simulink model "reaktor"  (R2016a)
settings: Solver=VariableStepAuto  StartTime=0.0  StopTime=100  RelTol=1e-3
values from neighbouring files (symbols this model uses):
  A_fm = 59900/3    (= 19966.6666667)    [zmienne.m]
  alfa_c = -2.0 * 10^-4    (= -0.0002)    [zmienne.m]
  alfa_f = -1.1 * 10^-5    (= -1.1e-05)    [zmienne.m]
  B_1 = 0.000209    [zmienne.m]
  B_2 = 0.001414    [zmienne.m]
  B_3 = 0.001309    [zmienne.m]
  B_4 = 0.002727    [zmienne.m]
  B_5 = 0.000925    [zmienne.m]
  B_6 = 0.000314    [zmienne.m]
  B_t = 0.00689    [zmienne.m]
  C_pf = 0.059    [zmienne.m]
  C_pmo = 1.39    [zmienne.m]
  CP_fw = 1.218    [zmienne.m]
  F_r = 0.974    [zmienne.m]
  H_fm = 200/3600    (= 0.0555555555556)    [zmienne.m]
  K9 = -0.035    [zmienne.m]
  lambda_1 = 0.0125    [zmienne.m]
  lambda_2 = 0.0308    [zmienne.m]
  lambda_3 = 0.114    [zmienne.m]
  lambda_4 = 0.307    [zmienne.m]
  lambda_5 = 1.19    [zmienne.m]
  lambda_6 = 3.19    [zmienne.m]
  M_f = M_ft * 3    (= 668217)    [zmienne.m]
  M_mo = V_mo * DENS_mo / 3    (= 8227.8)    [zmienne.m]
  NGT = 17.9 * 10^-6    (= 1.79e-05)    [zmienne.m]
  P_0 = (P_cor10 * 3.41) / (3600 * 3)    (= 1084885.18519)    [zmienne.m]
  POWER_i = 691244.4199    [zmienne.m]
  T_f10 = 1488.75    [zmienne.m]
  T_f20 = 1506.38    [zmienne.m]
  T_f30 = 1523.96    [zmienne.m]
  T_mo10 = 548.303    [zmienne.m]
  T_mo20 = 557.106    [zmienne.m]
  T_mo30 = 565.909    [zmienne.m]
  T_mo40 = 574.711    [zmienne.m]
  T_mo50 = 583.514    [zmienne.m]
  T_mo60 = 592.5    [zmienne.m]
  tau_cl = M_cl / W_pt    (= 2.08881752232)    [zmienne.m]
  tau_hl = M_hl / W_pt    (= 1.04440876116)    [zmienne.m]
  tau_la1 = 10    [zmienne.m]
  tau_la2 = 5    [zmienne.m]
  tau_le = 80    [zmienne.m]
  tau_lp = M_lp / W_pt    (= 1.87053609124)    [zmienne.m]
  tau_mo = M_mo / (2 * W_pt)    (= 0.0939967885046)    [zmienne.m]
  tau_rtd = 4    [zmienne.m]
  tau_set = 30    [zmienne.m]
  tau_up = M_up / W_pt    (= 1.43710645536)    [zmienne.m]
  X8 = 1225.85    [zmienne.m]
settings Model: Creator=Użytkownik  LastModifiedBy=Użytkownik
settings GRTTargetCC: GeneratePreprocessorConditionals=Use local settings

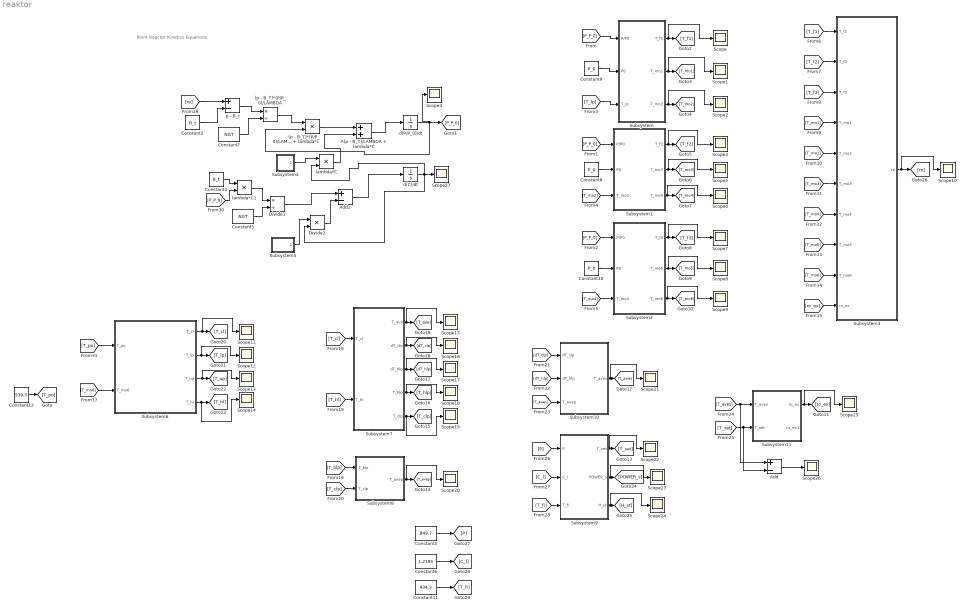
== system reaktor ==
  note: Point Reactor Kinetics Equations
  (p - B_T)*(P/P_0)/LAMBDA : Product  Inputs=*/
  (p - B_T)*(P/P_0)/LAMBDA + lambda*c : Product  Inputs=**
  A(p - B_T)/LAMBDA + lambda*C : Sum
  Add : Sum  Inputs=+-
  Add1 : Sum  Inputs=+-
  Constant10 : Constant  Value=P_0
  Constant11 : Constant  Value=434.3
  Constant12 : Constant  Value=539.5
  Constant2 : Constant  Value=B_t
  Constant3 : Constant  Value=849.7
  Constant4 : Constant  Value=B_t
  Constant5 : Constant  Value=NGT
  Constant6 : Constant  Value=1.2195
  Constant7 : Constant  Value=NGT
  Constant8 : Constant  Value=P_0
  Constant9 : Constant  Value=P_0
  Divide1 : Product  Inputs=*/
  Divide2 : Product  Inputs=**
  Scope{,1..27} (28 alike) : Scope
  Subsystem : Subsystem
  Subsystem1 : Subsystem
  Subsystem10 : Subsystem
  Subsystem11 : Subsystem
  Subsystem2 : Subsystem
  Subsystem3 : Subsystem
  Subsystem4 : Subsystem
  Subsystem5 : Subsystem
  Subsystem6 : Subsystem
  Subsystem7 : Subsystem
  Subsystem8 : Subsystem
  Subsystem9 : Subsystem
  d(C)/dt : Integrator  InitialCondition=4625.71
  d(P/P_0)/dt : Integrator  InitialCondition=1
  lambda*C : Product  Inputs=**
  lambda*C1 : Product  Inputs=**
  p - B_t : Sum  Inputs=+-
  wires:
  Constant2/1 -> p - B_t/2
  p - B_t/1 -> (p - B_T)*(P/P_0)/LAMBDA/1
  Constant7/1 -> (p - B_T)*(P/P_0)/LAMBDA/2
  Subsystem4/1(lambda) -> lambda*C/1
  d(C)/dt/1 -> Scope27/1, Divide2/2, lambda*C/2
  lambda*C/1 -> A(p - B_T)/LAMBDA + lambda*C/2
  A(p - B_T)/LAMBDA + lambda*C/1 -> d(P/P_0)/dt/1
  Constant5/1 -> Divide1/2
  (p - B_T)*(P/P_0)/LAMBDA/1 -> (p - B_T)*(P/P_0)/LAMBDA + lambda*c/1
  (p - B_T)*(P/P_0)/LAMBDA + lambda*c/1 -> A(p - B_T)/LAMBDA + lambda*C/1
  Divide1/1 -> Add1/1
  Subsystem5/1(lambda) -> Divide2/1
  Divide2/1 -> Add1/2
  Add1/1 -> d(C)/dt/1
  d(P/P_0)/dt/1 -> (p - B_T)*(P/P_0)/LAMBDA + lambda*c/2, [P_P_0], Scope4/1
  Constant9/1 -> Subsystem/2(P0)
  Constant8/1 -> Subsystem1/2(P0)
  Constant10/1 -> Subsystem2/2(P0)
  [T_po] -> Subsystem6/1(T_po)
  [P_P_0] -> Subsystem/1("P/P0 ")
  [P_P_0] -> Subsystem1/1("P/P0 ")
  [P_P_0] -> Subsystem2/1("P/P0 ")
  Subsystem/1(T_f1) -> Scope/1, [T_f1]
  Subsystem/2(T_mo1) -> Scope1/1, [T_mo1]
  Subsystem/3(T_mo2) -> Scope2/1, [T_mo2]
  Subsystem1/1(T_f2) -> Scope3/1, [T_f2]
  Subsystem1/2(T_mo3) -> Scope5/1, [T_mo3]
  Subsystem1/3(T_mo4) -> Scope6/1, [T_mo4]
  Subsystem2/1(T_f3) -> Scope7/1, [T_f3]
  Subsystem2/2(T_mo5) -> Scope8/1, [T_mo5]
  Subsystem2/3(T_mo6) -> Scope9/1, [T_mo6]
  [T_lp] -> Subsystem/3(T_lp)
  [T_mo2] -> Subsystem1/3(T_mo2)
  [T_mo4] -> Subsystem2/3(T_mo4)
  [T_f1] -> Subsystem3/1(T_f1)
  [T_f2] -> Subsystem3/2(T_f2)
  [T_f3] -> Subsystem3/3(T_f3)
  [T_mo1] -> Subsystem3/4(T_mo1)
  [T_mo2] -> Subsystem3/5(T_mo2)
  [T_mo3] -> Subsystem3/6(T_mo3)
  [T_mo4] -> Subsystem3/7(T_mo4)
  [T_mo5] -> Subsystem3/8(T_mo5)
  [T_mo6] -> Subsystem3/9(T_mo6)
  [ro_ex] -> Subsystem3/10(ro_ex)
  [T_cl] -> Subsystem7/1(T_cl)
  [T_hl] -> Subsystem7/2(T_hl)
  [T_hlp] -> Subsystem8/1(T_hlp)
  [T_clp] -> Subsystem8/2(T_clp)
  [dT_clp] -> Subsystem10/1(dT_clp)
  [dT_hlp] -> Subsystem10/2(dT_hlp)
  [T_avep] -> Subsystem10/3(T_avep)
  [T_aves] -> Add/1, Subsystem11/1(T_aves)
  [T_set] -> Add/2, Subsystem11/2(T_set)
  Subsystem10/1(T_aves) -> Scope21/1, [T_aves]
  Subsystem9/1(T_set) -> Scope22/1, [T_set]
  Subsystem8/1(T_avep) -> Scope20/1, [T_avep]
  Subsystem7/5(T_clp) -> Scope19/1, [T_clp]
  Subsystem7/4(T_hlp) -> Scope18/1, [T_hlp]
  Subsystem7/3(dT_hlp) -> Scope17/1, [dT_hlp]
  Subsystem7/2(dT_clp) -> Scope16/1, [dT_clp]
  Subsystem7/1(T_ave) -> Scope15/1, [T_ave]
  Subsystem6/3(T_up) -> Scope13/1, [T_up]
  Subsystem6/2(T_lp) -> Scope12/1, [T_lp]
  Subsystem6/1(T_cl) -> Scope11/1, [T_cl]
  Subsystem9/2(POWER_s) -> [POWER_s], Scope23/1
  [P] -> Subsystem9/1(P)
  [C_l] -> Subsystem9/2(C_l)
  [T_fi] -> Subsystem9/3(T_fi)
  [T_mo6] -> Subsystem6/2(T_mo6)
  Subsystem3/1(ro) -> Scope10/1, [ro]
  Constant3/1 -> [P]
  Constant6/1 -> [C_l]
  Constant4/1 -> lambda*C1/1
  [P_P_0] -> lambda*C1/2
  lambda*C1/1 -> Divide1/1
  Subsystem11/1(ro_ex) -> Scope25/1, [ro_ex]
  Subsystem9/3(H_st) -> Scope24/1, [H_st]
  Add/1 -> Scope26/1
  Subsystem6/4(T_hl) -> Scope14/1, [T_hl]
  Constant11/1 -> [T_fi]
  Constant12/1 -> [T_po]
  [ro] -> p - B_t/1

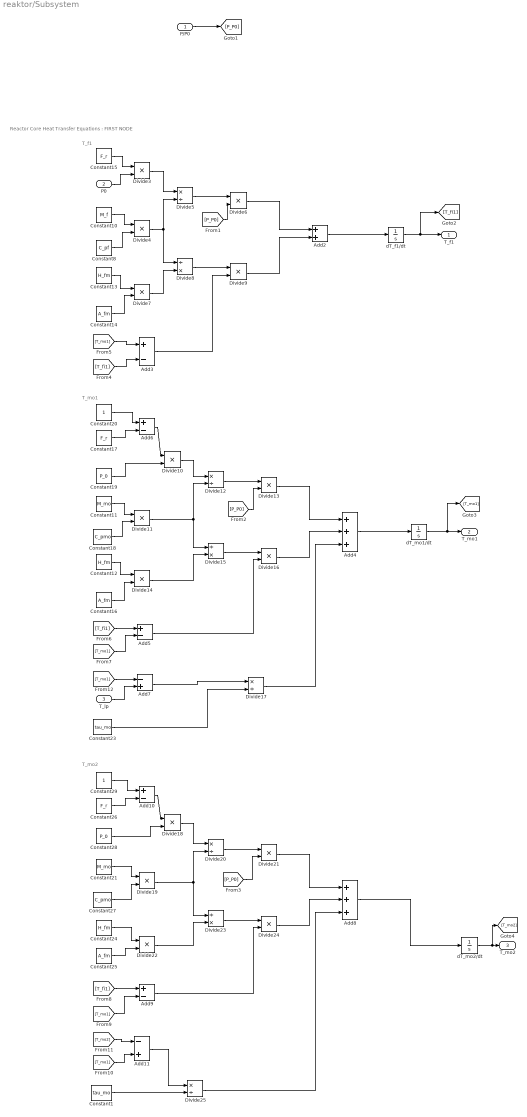
== system reaktor/Subsystem ==
  note: T_mo2
  note: T_mo1
  note: T_f1
  note: Reactor Core Heat Transfer Equations : FIRST NODE
  "P/P0 " : Inport
  P0 : Inport  Port=2
  T_lp : Inport  Port=3
  Add{3,5..6,9..10} (5 alike) : Sum  Inputs=+-
  Add11 : Sum  Inputs=-+
  Add2 : Sum
  Add4 : Sum  Inputs=+++
  Add7 : Sum  Inputs=-+
  Add8 : Sum  Inputs=+++
  Constant1 : Constant  Value=tau_mo
  Constant10 : Constant  Value=M_f
  Constant11 : Constant  Value=M_mo
  Constant12 : Constant  Value=H_fm
  Constant13 : Constant  Value=H_fm
  Constant14 : Constant  Value=A_fm
  Constant15 : Constant  Value=F_r
  Constant16 : Constant  Value=A_fm
  Constant17 : Constant  Value=F_r
  Constant18 : Constant  Value=C_pmo
  Constant19 : Constant  Value=P_0
  Constant20 : Constant
  Constant21 : Constant  Value=M_mo
  Constant23 : Constant  Value=tau_mo
  Constant24 : Constant  Value=H_fm
  Constant25 : Constant  Value=A_fm
  Constant26 : Constant  Value=F_r
  Constant27 : Constant  Value=C_pmo
  Constant28 : Constant  Value=P_0
  Constant29 : Constant
  Constant8 : Constant  Value=C_pf
  Divide{3..4,6..7,9..11,13..14,16,18..19,21..22,24} (15 alike) : Product  Inputs=**
  Divide{5,12,17,20,25} (5 alike) : Product  Inputs=*/
  Divide15 : Product  Inputs=/*
  Divide23 : Product  Inputs=/*
  Divide8 : Product  Inputs=/*
  dT_f1/dt : Integrator  InitialCondition=1488.75
  dT_mo1/dt : Integrator  InitialCondition=548.303
  dT_mo2/dt : Integrator  InitialCondition=557.106
  T_f1 : Outport
  T_mo1 : Outport  Port=2
  T_mo2 : Outport  Port=3
  wires:
  Constant15/1 -> Divide3/1
  Constant10/1 -> Divide4/1
  Constant8/1 -> Divide4/2
  Divide3/1 -> Divide5/1
  Divide4/1 -> Divide5/2, Divide8/1
  Divide5/1 -> Divide6/1
  Divide6/1 -> Add2/1
  Constant13/1 -> Divide7/1
  Constant14/1 -> Divide7/2
  Divide7/1 -> Divide8/2
  Divide8/1 -> Divide9/1
  dT_mo1/dt/1 -> [T_mo1], T_mo1/1
  dT_f1/dt/1 -> [T_fi1], T_f1/1
  Add3/1 -> Divide9/2
  Divide9/1 -> Add2/2
  Add2/1 -> dT_f1/dt/1
  Constant19/1 -> Divide10/2
  Constant11/1 -> Divide11/1
  Constant18/1 -> Divide11/2
  Divide10/1 -> Divide12/1
  Divide11/1 -> Divide15/1, Divide12/2
  Divide12/1 -> Divide13/1
  Divide13/1 -> Add4/1
  Constant12/1 -> Divide14/1
  Constant16/1 -> Divide14/2
  Divide14/1 -> Divide15/2
  Divide15/1 -> Divide16/1
  Add5/1 -> Divide16/2
  Divide16/1 -> Add4/2
  Constant20/1 -> Add6/1
  Constant17/1 -> Add6/2
  Add6/1 -> Divide10/1
  T_lp/1 -> Add7/2
  Add7/1 -> Divide17/1
  Constant23/1 -> Divide17/2
  Divide17/1 -> Add4/3
  Add4/1 -> dT_mo1/dt/1
  dT_mo2/dt/1 -> [T_mo2], T_mo2/1
  Constant28/1 -> Divide18/2
  Constant21/1 -> Divide19/1
  Constant27/1 -> Divide19/2
  Divide18/1 -> Divide20/1
  Divide19/1 -> Divide20/2, Divide23/1
  Divide20/1 -> Divide21/1
  Divide21/1 -> Add8/1
  Constant24/1 -> Divide22/1
  Constant25/1 -> Divide22/2
  Divide22/1 -> Divide23/2
  Divide23/1 -> Divide24/1
  Add9/1 -> Divide24/2
  Divide24/1 -> Add8/2
  Constant29/1 -> Add10/1
  Constant26/1 -> Add10/2
  Add10/1 -> Divide18/1
  Add11/1 -> Divide25/1
  Divide25/1 -> Add8/3
  Add8/1 -> dT_mo2/dt/1
  "P/P0 "/1 -> [P_P0]
  P0/1 -> Divide3/2
  [P_P0] -> Divide6/2
  [P_P0] -> Divide21/2
  [P_P0] -> Divide13/2
  [T_mo1] -> Add3/1
  [T_fi1] -> Add3/2
  [T_fi1] -> Add5/1
  [T_mo1] -> Add5/2
  [T_fi1] -> Add9/1
  [T_mo1] -> Add9/2
  [T_mo2] -> Add11/1
  [T_mo1] -> Add11/2
  [T_mo1] -> Add7/1
  Constant1/1 -> Divide25/2

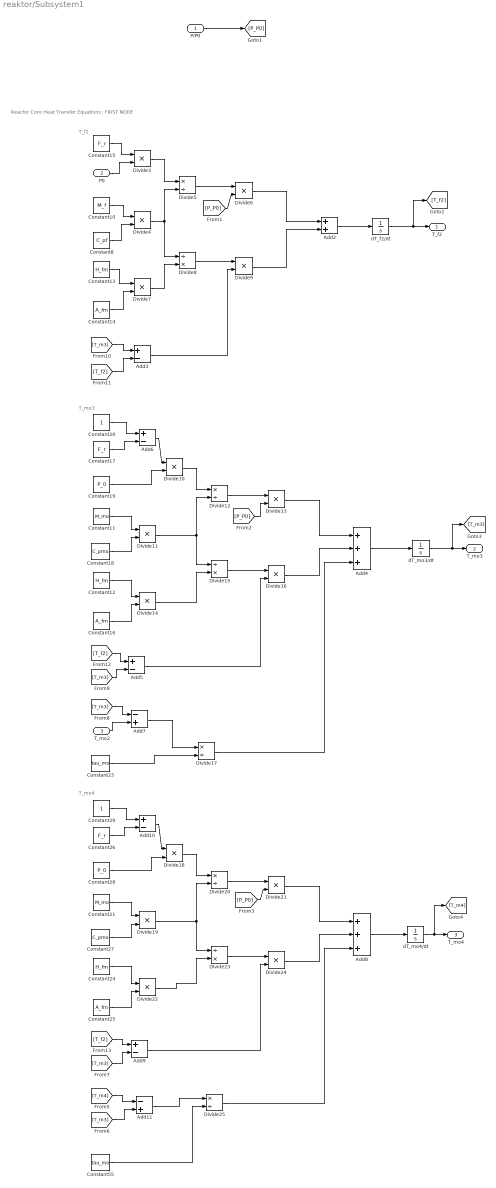
== system reaktor/Subsystem1 ==
  note: T_mo4
  note: T_mo3
  note: T_f2
  note: Reactor Core Heat Transfer Equations : FIRST NODE
  "P/P0 " : Inport
  P0 : Inport  Port=2
  T_mo2 : Inport  Port=3
  Add{3,5..6,9..10} (5 alike) : Sum  Inputs=+-
  Add11 : Sum  Inputs=-+
  Add2 : Sum
  Add4 : Sum  Inputs=+++
  Add7 : Sum  Inputs=-+
  Add8 : Sum  Inputs=+++
  Constant10 : Constant  Value=M_f
  Constant11 : Constant  Value=M_mo
  Constant12 : Constant  Value=H_fm
  Constant13 : Constant  Value=H_fm
  Constant14 : Constant  Value=A_fm
  Constant15 : Constant  Value=F_r
  Constant16 : Constant  Value=A_fm
  Constant17 : Constant  Value=F_r
  Constant18 : Constant  Value=C_pmo
  Constant19 : Constant  Value=P_0
  Constant20 : Constant
  Constant21 : Constant  Value=M_mo
  Constant23 : Constant  Value=tau_mo
  Constant24 : Constant  Value=H_fm
  Constant25 : Constant  Value=A_fm
  Constant26 : Constant  Value=F_r
  Constant27 : Constant  Value=C_pmo
  Constant28 : Constant  Value=P_0
  Constant29 : Constant
  Constant55 : Constant  Value=tau_mo
  Constant8 : Constant  Value=C_pf
  Divide{3..4,6..7,9..11,13..14,16,18..19,21..22,24} (15 alike) : Product  Inputs=**
  Divide{5,12,17,20,25} (5 alike) : Product  Inputs=*/
  Divide15 : Product  Inputs=/*
  Divide23 : Product  Inputs=/*
  Divide8 : Product  Inputs=/*
  dT_f2/dt : Integrator  InitialCondition=1506.38
  dT_mo3/dt : Integrator  InitialCondition=565.90
  dT_mo4/dt : Integrator  InitialCondition=574.711
  T_f2 : Outport
  T_mo3 : Outport  Port=2
  T_mo4 : Outport  Port=3
  wires:
  Constant15/1 -> Divide3/1
  Constant10/1 -> Divide4/1
  Constant8/1 -> Divide4/2
  Divide3/1 -> Divide5/1
  Divide4/1 -> Divide5/2, Divide8/1
  Divide5/1 -> Divide6/1
  Divide6/1 -> Add2/1
  Constant13/1 -> Divide7/1
  Constant14/1 -> Divide7/2
  Divide7/1 -> Divide8/2
  Divide8/1 -> Divide9/1
  dT_mo3/dt/1 -> [T_m3], T_mo3/1
  dT_f2/dt/1 -> [T_f2], T_f2/1
  Add3/1 -> Divide9/2
  Divide9/1 -> Add2/2
  Add2/1 -> dT_f2/dt/1
  Constant19/1 -> Divide10/2
  Constant11/1 -> Divide11/1
  Constant18/1 -> Divide11/2
  Divide10/1 -> Divide12/1
  Divide11/1 -> Divide12/2, Divide15/1
  Divide12/1 -> Divide13/1
  Divide13/1 -> Add4/1
  Constant12/1 -> Divide14/1
  Constant16/1 -> Divide14/2
  Divide14/1 -> Divide15/2
  Divide15/1 -> Divide16/1
  Add5/1 -> Divide16/2
  Divide16/1 -> Add4/2
  Constant20/1 -> Add6/1
  Constant17/1 -> Add6/2
  Add6/1 -> Divide10/1
  T_mo2/1 -> Add7/2
  Add7/1 -> Divide17/1
  Constant23/1 -> Divide17/2
  Divide17/1 -> Add4/3
  Add4/1 -> dT_mo3/dt/1
  dT_mo4/dt/1 -> T_mo4/1, [T_m4]
  Constant28/1 -> Divide18/2
  Constant21/1 -> Divide19/1
  Constant27/1 -> Divide19/2
  Divide18/1 -> Divide20/1
  Divide19/1 -> Divide20/2, Divide23/1
  Divide20/1 -> Divide21/1
  Divide21/1 -> Add8/1
  Constant24/1 -> Divide22/1
  Constant25/1 -> Divide22/2
  Divide22/1 -> Divide23/2
  Divide23/1 -> Divide24/1
  Add9/1 -> Divide24/2
  Divide24/1 -> Add8/2
  Constant29/1 -> Add10/1
  Constant26/1 -> Add10/2
  Add10/1 -> Divide18/1
  Add11/1 -> Divide25/1
  Divide25/1 -> Add8/3
  Add8/1 -> dT_mo4/dt/1
  "P/P0 "/1 -> [P_P0]
  P0/1 -> Divide3/2
  [P_P0] -> Divide21/2
  [P_P0] -> Divide13/2
  [P_P0] -> Divide6/2
  [T_m3] -> Add11/2
  [T_m3] -> Add9/2
  [T_m3] -> Add7/1
  [T_m3] -> Add5/2
  [T_m3] -> Add3/1
  [T_f2] -> Add3/2
  [T_f2] -> Add5/1
  [T_f2] -> Add9/1
  [T_m4] -> Add11/1
  Constant55/1 -> Divide25/2

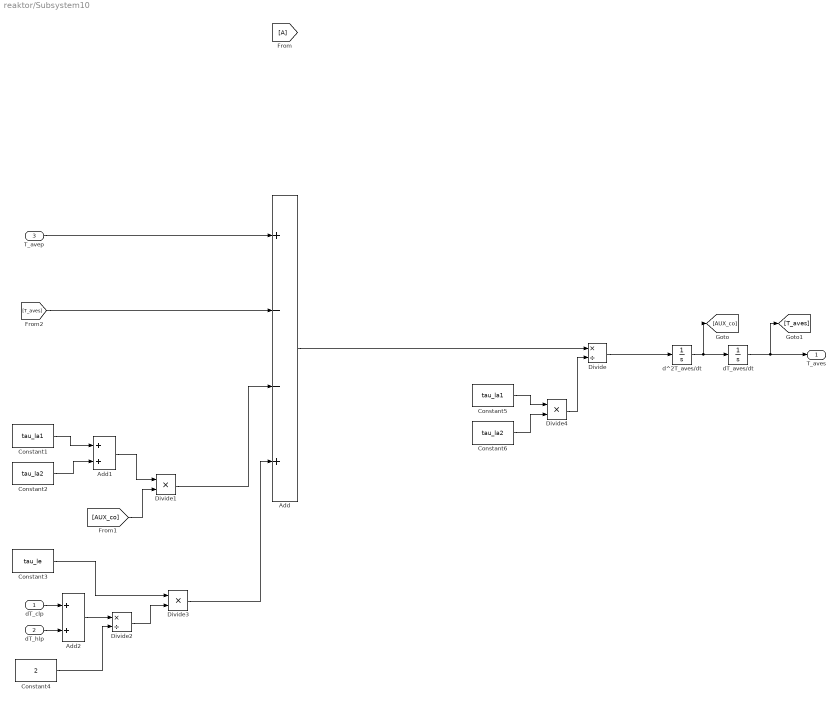
== system reaktor/Subsystem10 ==
  dT_clp : Inport
  dT_hlp : Inport  Port=2
  T_avep : Inport  Port=3
  Add : Sum  Inputs=+--+
  Add1 : Sum
  Add2 : Sum
  Constant1 : Constant  Value=tau_la1
  Constant2 : Constant  Value=tau_la2
  Constant3 : Constant  Value=tau_le
  Constant4 : Constant  Value=2
  Constant5 : Constant  Value=tau_la1
  Constant6 : Constant  Value=tau_la2
  Divide : Product  Inputs=*/
  Divide1 : Product  Inputs=**
  Divide2 : Product  Inputs=*/
  Divide3 : Product  Inputs=**
  Divide4 : Product  Inputs=**
  dT_aves/dt : Integrator  InitialCondition=566
  d^2T_aves/dt : Integrator
  T_aves : Outport
  wires:
  T_avep/1 -> Add/1
  dT_aves/dt/1 -> [T_aves], T_aves/1
  Constant1/1 -> Add1/1
  Constant2/1 -> Add1/2
  Add1/1 -> Divide1/1
  d^2T_aves/dt/1 -> [AUX_co], dT_aves/dt/1
  Divide1/1 -> Add/3
  dT_clp/1 -> Add2/1
  dT_hlp/1 -> Add2/2
  Add2/1 -> Divide2/1
  Constant4/1 -> Divide2/2
  Constant3/1 -> Divide3/1
  Divide2/1 -> Divide3/2
  Divide3/1 -> Add/4
  Constant5/1 -> Divide4/1
  Constant6/1 -> Divide4/2
  Divide4/1 -> Divide/2
  Add/1 -> Divide/1
  Divide/1 -> d^2T_aves/dt/1
  [AUX_co] -> Divide1/2
  [T_aves] -> Add/2

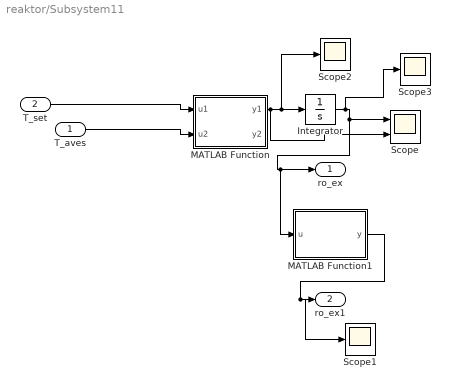
== system reaktor/Subsystem11 ==
  T_aves : Inport
  T_set : Inport  Port=2
  Integrator : Integrator
  MATLAB Function : MATLAB Function  TreatAsAtomicUnit=on
  MATLAB Function1 : MATLAB Function  TreatAsAtomicUnit=on
  Scope : Scope  NumInputPorts=2
  Scope1 : Scope
  Scope2 : Scope
  Scope3 : Scope
  ro_ex : Outport
  ro_ex1 : Outport  Port=2
  wires:
  T_set/1 -> MATLAB Function/1(u1)
  T_aves/1 -> MATLAB Function/2(u2)
  MATLAB Function/1(y1) -> Scope/2, Scope2/1, Integrator/1
  Integrator/1 -> Scope3/1, MATLAB Function1/1(u), ro_ex/1, Scope/1
  MATLAB Function1/1(y) -> Scope1/1, ro_ex1/1

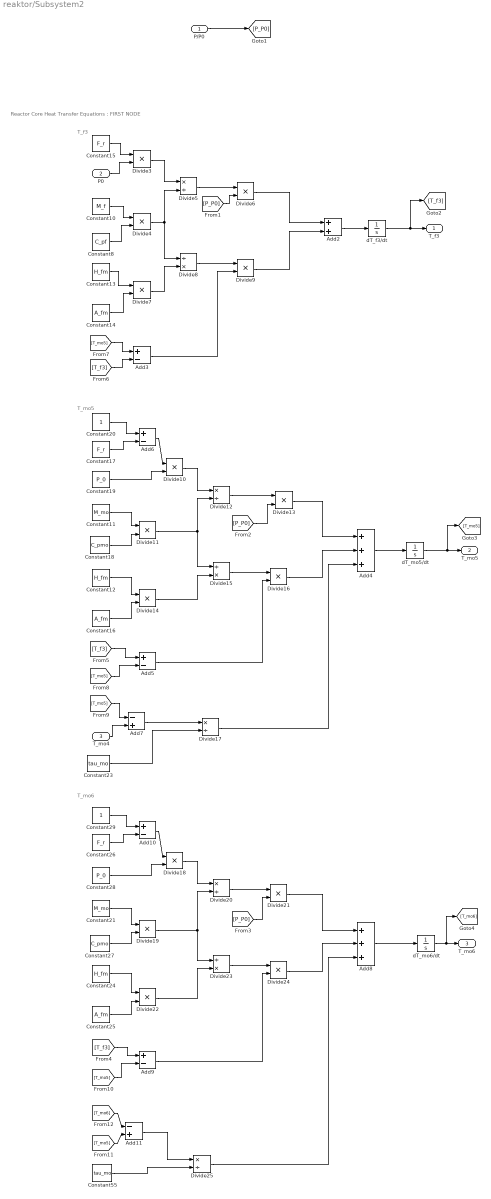
== system reaktor/Subsystem2 ==
  note: T_mo6
  note: T_mo5
  note: T_f3
  note: Reactor Core Heat Transfer Equations : FIRST NODE
  "P/P0 " : Inport
  P0 : Inport  Port=2
  T_mo4 : Inport  Port=3
  Add{3,5..6,9..10} (5 alike) : Sum  Inputs=+-
  Add11 : Sum  Inputs=-+
  Add2 : Sum
  Add4 : Sum  Inputs=+++
  Add7 : Sum  Inputs=-+
  Add8 : Sum  Inputs=+++
  Constant10 : Constant  Value=M_f
  Constant11 : Constant  Value=M_mo
  Constant12 : Constant  Value=H_fm
  Constant13 : Constant  Value=H_fm
  Constant14 : Constant  Value=A_fm
  Constant15 : Constant  Value=F_r
  Constant16 : Constant  Value=A_fm
  Constant17 : Constant  Value=F_r
  Constant18 : Constant  Value=C_pmo
  Constant19 : Constant  Value=P_0
  Constant20 : Constant
  Constant21 : Constant  Value=M_mo
  Constant23 : Constant  Value=tau_mo
  Constant24 : Constant  Value=H_fm
  Constant25 : Constant  Value=A_fm
  Constant26 : Constant  Value=F_r
  Constant27 : Constant  Value=C_pmo
  Constant28 : Constant  Value=P_0
  Constant29 : Constant
  Constant55 : Constant  Value=tau_mo
  Constant8 : Constant  Value=C_pf
  Divide{3..4,6..7,9..11,13..14,16,18..19,21..22,24} (15 alike) : Product  Inputs=**
  Divide{5,12,17,20,25} (5 alike) : Product  Inputs=*/
  Divide15 : Product  Inputs=/*
  Divide23 : Product  Inputs=/*
  Divide8 : Product  Inputs=/*
  dT_f3/dt : Integrator  InitialCondition=1523.96
  dT_mo5/dt : Integrator  InitialCondition=583.514
  dT_mo6/dt : Integrator  InitialCondition=592.5
  T_f3 : Outport
  T_mo5 : Outport  Port=2
  T_mo6 : Outport  Port=3
  wires:
  Constant15/1 -> Divide3/1
  Constant10/1 -> Divide4/1
  Constant8/1 -> Divide4/2
  Divide3/1 -> Divide5/1
  Divide4/1 -> Divide5/2, Divide8/1
  Divide5/1 -> Divide6/1
  Divide6/1 -> Add2/1
  Constant13/1 -> Divide7/1
  Constant14/1 -> Divide7/2
  Divide7/1 -> Divide8/2
  Divide8/1 -> Divide9/1
  dT_mo5/dt/1 -> [T_mo5], T_mo5/1
  dT_f3/dt/1 -> [T_f3], T_f3/1
  Add3/1 -> Divide9/2
  Divide9/1 -> Add2/2
  Add2/1 -> dT_f3/dt/1
  Constant19/1 -> Divide10/2
  Constant11/1 -> Divide11/1
  Constant18/1 -> Divide11/2
  Divide10/1 -> Divide12/1
  Divide11/1 -> Divide15/1, Divide12/2
  Divide12/1 -> Divide13/1
  Divide13/1 -> Add4/1
  Constant12/1 -> Divide14/1
  Constant16/1 -> Divide14/2
  Divide14/1 -> Divide15/2
  Divide15/1 -> Divide16/1
  Add5/1 -> Divide16/2
  Divide16/1 -> Add4/2
  Constant20/1 -> Add6/1
  Constant17/1 -> Add6/2
  Add6/1 -> Divide10/1
  T_mo4/1 -> Add7/2
  Add7/1 -> Divide17/1
  Constant23/1 -> Divide17/2
  Divide17/1 -> Add4/3
  Add4/1 -> dT_mo5/dt/1
  Constant28/1 -> Divide18/2
  Constant21/1 -> Divide19/1
  Constant27/1 -> Divide19/2
  Divide18/1 -> Divide20/1
  Divide19/1 -> Divide20/2, Divide23/1
  Divide20/1 -> Divide21/1
  Divide21/1 -> Add8/1
  Constant24/1 -> Divide22/1
  Constant25/1 -> Divide22/2
  Divide22/1 -> Divide23/2
  Divide23/1 -> Divide24/1
  Add9/1 -> Divide24/2
  Divide24/1 -> Add8/2
  Constant29/1 -> Add10/1
  Constant26/1 -> Add10/2
  Add10/1 -> Divide18/1
  Add11/1 -> Divide25/1
  Divide25/1 -> Add8/3
  Add8/1 -> dT_mo6/dt/1
  Constant55/1 -> Divide25/2
  "P/P0 "/1 -> [P_P0]
  P0/1 -> Divide3/2
  [P_P0] -> Divide21/2
  [P_P0] -> Divide13/2
  [P_P0] -> Divide6/2
  [T_f3] -> Add9/1
  [T_f3] -> Add5/1
  [T_f3] -> Add3/2
  [T_mo5] -> Add3/1
  [T_mo5] -> Add5/2
  [T_mo5] -> Add7/1
  [T_mo5] -> Add9/2
  [T_mo5] -> Add11/2
  [T_mo6] -> Add11/1
  dT_mo6/dt/1 -> [T_mo6], T_mo6/1

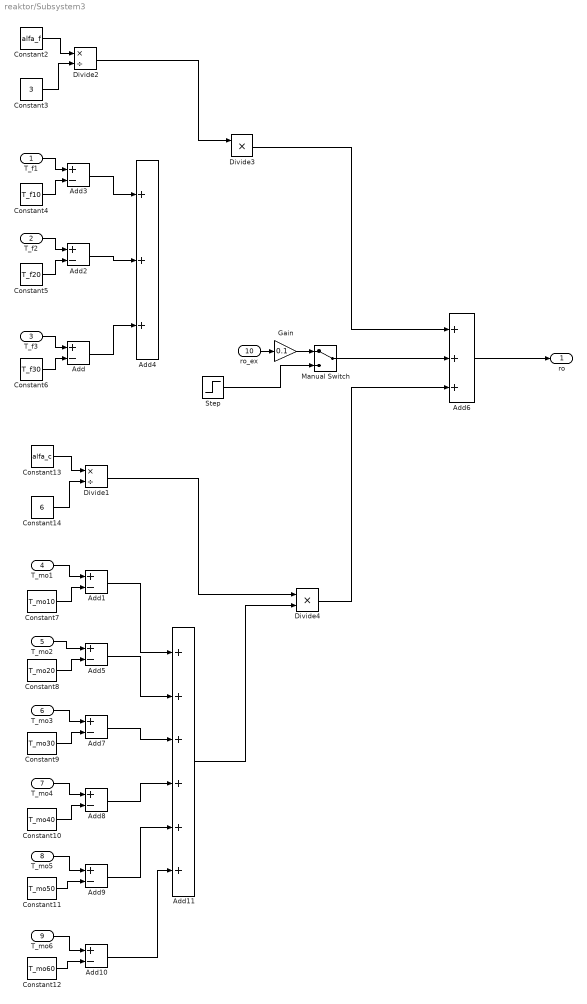
== system reaktor/Subsystem3 ==
  T_f1 : Inport
  T_f2 : Inport  Port=2
  T_f3 : Inport  Port=3
  T_mo1 : Inport  Port=4
  T_mo2 : Inport  Port=5
  T_mo3 : Inport  Port=6
  T_mo4 : Inport  Port=7
  T_mo5 : Inport  Port=8
  T_mo6 : Inport  Port=9
  ro_ex : Inport  Port=10
  Add{,1..3,5,7..10} (9 alike) : Sum  Inputs=+-
  Add11 : Sum  Inputs=6
  Add4 : Sum  Inputs=+++
  Add6 : Sum  Inputs=+++
  Constant10 : Constant  Value=T_mo40
  Constant11 : Constant  Value=T_mo50
  Constant12 : Constant  Value=T_mo60
  Constant13 : Constant  Value=alfa_c
  Constant14 : Constant  Value=6
  Constant2 : Constant  Value=alfa_f
  Constant3 : Constant  Value=3
  Constant4 : Constant  Value=T_f10
  Constant5 : Constant  Value=T_f20
  Constant6 : Constant  Value=T_f30
  Constant7 : Constant  Value=T_mo10
  Constant8 : Constant  Value=T_mo20
  Constant9 : Constant  Value=T_mo30
  Divide1 : Product  Inputs=*/
  Divide2 : Product  Inputs=*/
  Divide3 : Product  Inputs=**
  Divide4 : Product  Inputs=**
  Gain : Gain  Gain=0.1
  Manual Switch : ManualSwitch
  Step : Step  After=0.0  SampleTime=0
  ro : Outport
  wires:
  Constant2/1 -> Divide2/1
  Constant3/1 -> Divide2/2
  Constant13/1 -> Divide1/1
  Constant14/1 -> Divide1/2
  Divide2/1 -> Divide3/1
  Divide1/1 -> Divide4/1
  Divide3/1 -> Add6/1
  Divide4/1 -> Add6/3
  Add6/1 -> ro/1
  Manual Switch/1 -> Add6/2
  ro_ex/1 -> Gain/1
  Step/1 -> Manual Switch/2
  T_f3/1 -> Add/1
  Constant6/1 -> Add/2
  Constant5/1 -> Add2/2
  T_f2/1 -> Add2/1
  Constant4/1 -> Add3/2
  T_f1/1 -> Add3/1
  Add3/1 -> Add4/1
  Add2/1 -> Add4/2
  Add/1 -> Add4/3
  T_mo1/1 -> Add1/1
  Constant7/1 -> Add1/2
  T_mo2/1 -> Add5/1
  Constant8/1 -> Add5/2
  T_mo3/1 -> Add7/1
  Constant9/1 -> Add7/2
  T_mo4/1 -> Add8/1
  Constant10/1 -> Add8/2
  T_mo5/1 -> Add9/1
  Constant11/1 -> Add9/2
  T_mo6/1 -> Add10/1
  Constant12/1 -> Add10/2
  Add1/1 -> Add11/1
  Add5/1 -> Add11/2
  Add7/1 -> Add11/3
  Add8/1 -> Add11/4
  Add9/1 -> Add11/5
  Add10/1 -> Add11/6
  Add11/1 -> Divide4/2
  Gain/1 -> Manual Switch/1

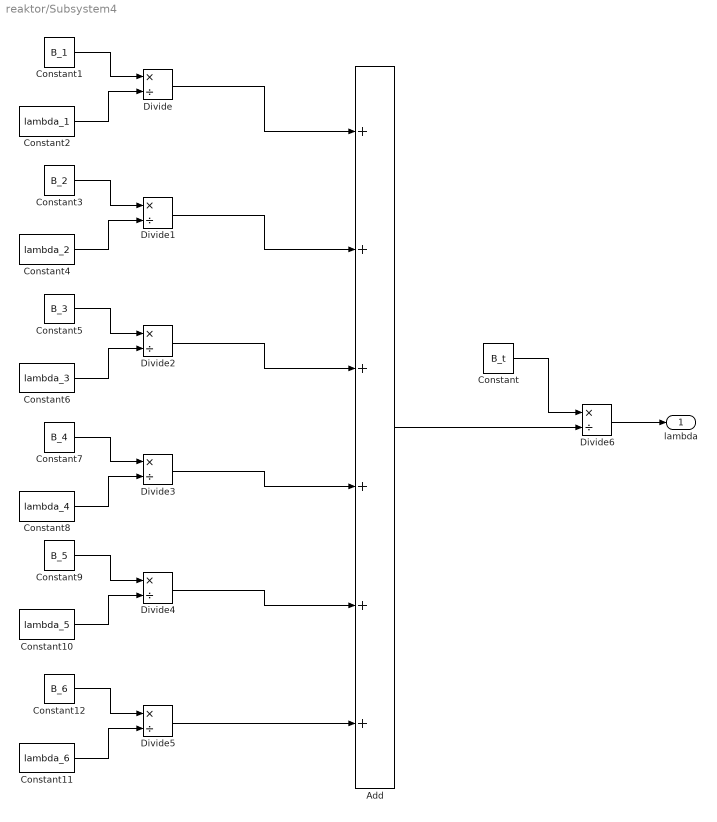
== system reaktor/Subsystem4 ==
  Add : Sum  Inputs=++++++
  Constant : Constant  Value=B_t
  Constant1 : Constant  Value=B_1
  Constant10 : Constant  Value=lambda_5
  Constant11 : Constant  Value=lambda_6
  Constant12 : Constant  Value=B_6
  Constant2 : Constant  Value=lambda_1
  Constant3 : Constant  Value=B_2
  Constant4 : Constant  Value=lambda_2
  Constant5 : Constant  Value=B_3
  Constant6 : Constant  Value=lambda_3
  Constant7 : Constant  Value=B_4
  Constant8 : Constant  Value=lambda_4
  Constant9 : Constant  Value=B_5
  Divide{,1..6} (7 alike) : Product  Inputs=*/
  lambda : Outport
  wires:
  Constant1/1 -> Divide/1
  Constant2/1 -> Divide/2
  Constant3/1 -> Divide1/1
  Constant4/1 -> Divide1/2
  Constant5/1 -> Divide2/1
  Constant6/1 -> Divide2/2
  Constant7/1 -> Divide3/1
  Constant8/1 -> Divide3/2
  Constant9/1 -> Divide4/1
  Constant10/1 -> Divide4/2
  Constant12/1 -> Divide5/1
  Constant11/1 -> Divide5/2
  Divide5/1 -> Add/6
  Divide4/1 -> Add/5
  Divide3/1 -> Add/4
  Divide1/1 -> Add/2
  Divide2/1 -> Add/3
  Divide/1 -> Add/1
  Add/1 -> Divide6/2
  Constant/1 -> Divide6/1
  Divide6/1 -> lambda/1

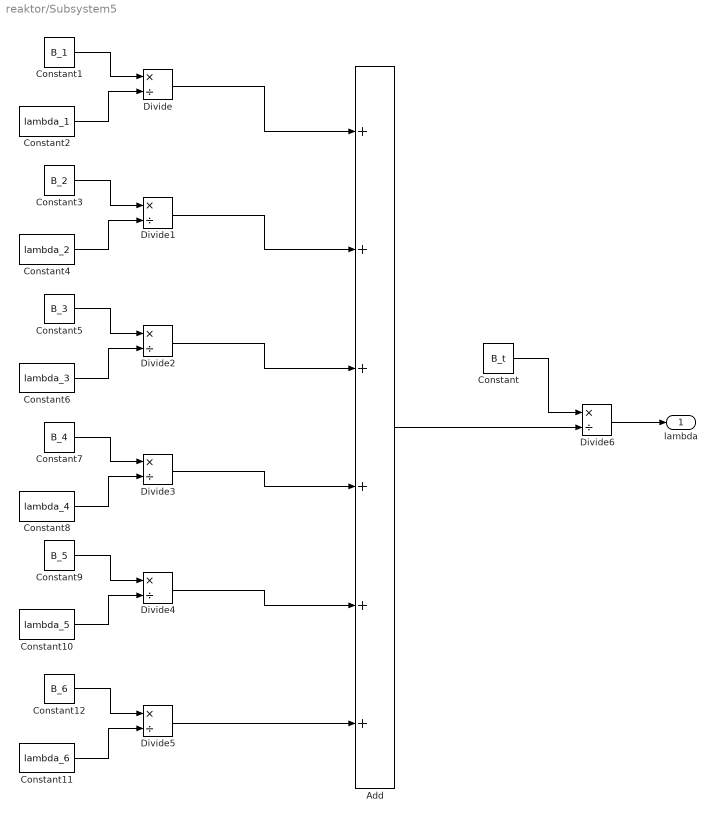
== system reaktor/Subsystem5 ==
  Add : Sum  Inputs=++++++
  Constant : Constant  Value=B_t
  Constant1 : Constant  Value=B_1
  Constant10 : Constant  Value=lambda_5
  Constant11 : Constant  Value=lambda_6
  Constant12 : Constant  Value=B_6
  Constant2 : Constant  Value=lambda_1
  Constant3 : Constant  Value=B_2
  Constant4 : Constant  Value=lambda_2
  Constant5 : Constant  Value=B_3
  Constant6 : Constant  Value=lambda_3
  Constant7 : Constant  Value=B_4
  Constant8 : Constant  Value=lambda_4
  Constant9 : Constant  Value=B_5
  Divide{,1..6} (7 alike) : Product  Inputs=*/
  lambda : Outport
  wires:
  Divide6/1 -> lambda/1
  Constant/1 -> Divide6/1
  Add/1 -> Divide6/2
  Divide/1 -> Add/1
  Divide2/1 -> Add/3
  Divide1/1 -> Add/2
  Divide3/1 -> Add/4
  Divide4/1 -> Add/5
  Divide5/1 -> Add/6
  Constant11/1 -> Divide5/2
  Constant12/1 -> Divide5/1
  Constant10/1 -> Divide4/2
  Constant9/1 -> Divide4/1
  Constant8/1 -> Divide3/2
  Constant7/1 -> Divide3/1
  Constant6/1 -> Divide2/2
  Constant5/1 -> Divide2/1
  Constant4/1 -> Divide1/2
  Constant3/1 -> Divide1/1
  Constant2/1 -> Divide/2
  Constant1/1 -> Divide/1

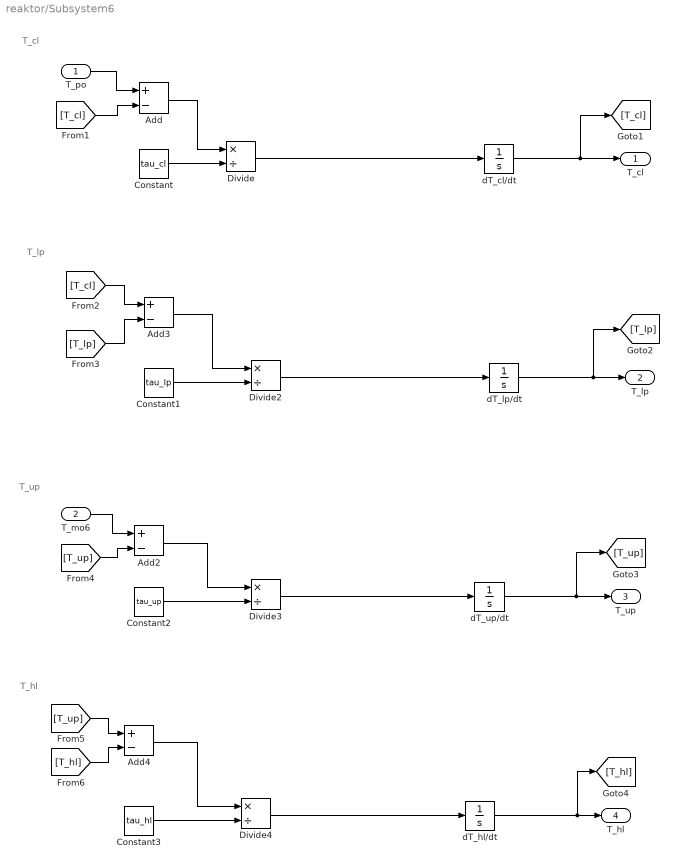
== system reaktor/Subsystem6 ==
  note: T_hl
  note: T_up
  note: T_lp
  note: T_cl
  T_po : Inport
  T_mo6 : Inport  Port=2
  Add{,2..4} (4 alike) : Sum  Inputs=+-
  Constant : Constant  Value=tau_cl
  Constant1 : Constant  Value=tau_lp
  Constant2 : Constant  Value=tau_up
  Constant3 : Constant  Value=tau_hl
  Divide{,2..4} (4 alike) : Product  Inputs=*/
  dT_cl/dt : Integrator  InitialCondition=539.5
  dT_hl/dt : Integrator  InitialCondition=592.5
  dT_lp/dt : Integrator  InitialCondition=539.5
  dT_up/dt : Integrator  InitialCondition=592.5
  T_cl : Outport
  T_lp : Outport  Port=2
  T_up : Outport  Port=3
  T_hl : Outport  Port=4
  wires:
  T_po/1 -> Add/1
  dT_cl/dt/1 -> [T_cl], T_cl/1
  Constant/1 -> Divide/2
  Add/1 -> Divide/1
  Divide/1 -> dT_cl/dt/1
  Constant2/1 -> Divide3/2
  Divide2/1 -> dT_lp/dt/1
  Divide3/1 -> dT_up/dt/1
  Divide4/1 -> dT_hl/dt/1
  dT_lp/dt/1 -> [T_lp], T_lp/1
  T_mo6/1 -> Add2/1
  Add2/1 -> Divide3/1
  dT_up/dt/1 -> [T_up], T_up/1
  dT_hl/dt/1 -> [T_hl], T_hl/1
  Add4/1 -> Divide4/1
  Constant1/1 -> Divide2/2
  Constant3/1 -> Divide4/2
  Add3/1 -> Divide2/1
  [T_cl] -> Add/2
  [T_cl] -> Add3/1
  [T_lp] -> Add3/2
  [T_up] -> Add2/2
  [T_up] -> Add4/1
  [T_hl] -> Add4/2

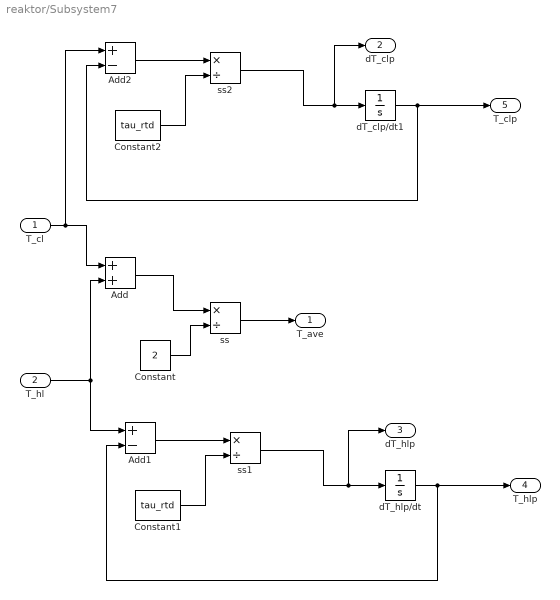
== system reaktor/Subsystem7 ==
  T_cl : Inport
  T_hl : Inport  Port=2
  Add : Sum
  Add1 : Sum  Inputs=+-
  Add2 : Sum  Inputs=+-
  Constant : Constant  Value=2
  Constant1 : Constant  Value=tau_rtd
  Constant2 : Constant  Value=tau_rtd
  dT_clp/dt1 : Integrator  InitialCondition=539.5
  dT_hlp/dt : Integrator  InitialCondition=592.5
  ss : Product  Inputs=*/
  ss1 : Product  Inputs=*/
  ss2 : Product  Inputs=*/
  T_ave : Outport
  dT_clp : Outport  Port=2
  dT_hlp : Outport  Port=3
  T_hlp : Outport  Port=4
  T_clp : Outport  Port=5
  wires:
  T_hl/1 -> Add1/1, Add/2
  Add/1 -> ss/1
  Constant/1 -> ss/2
  ss/1 -> T_ave/1
  dT_hlp/dt/1 -> Add1/2, T_hlp/1
  Add1/1 -> ss1/1
  Constant1/1 -> ss1/2
  ss1/1 -> dT_hlp/1, dT_hlp/dt/1
  T_cl/1 -> Add2/1, Add/1
  dT_clp/dt1/1 -> Add2/2, T_clp/1
  Add2/1 -> ss2/1
  Constant2/1 -> ss2/2
  ss2/1 -> dT_clp/1, dT_clp/dt1/1

== system reaktor/Subsystem8 ==
  T_hlp : Inport
  T_clp : Inport  Port=2
  Add1 : Sum
  Constant4 : Constant  Value=2
  Divide1 : Product  Inputs=*/
  T_avep : Outport
  wires:
  T_hlp/1 -> Add1/1
  T_clp/1 -> Add1/2
  Add1/1 -> Divide1/1
  Constant4/1 -> Divide1/2
  Divide1/1 -> T_avep/1

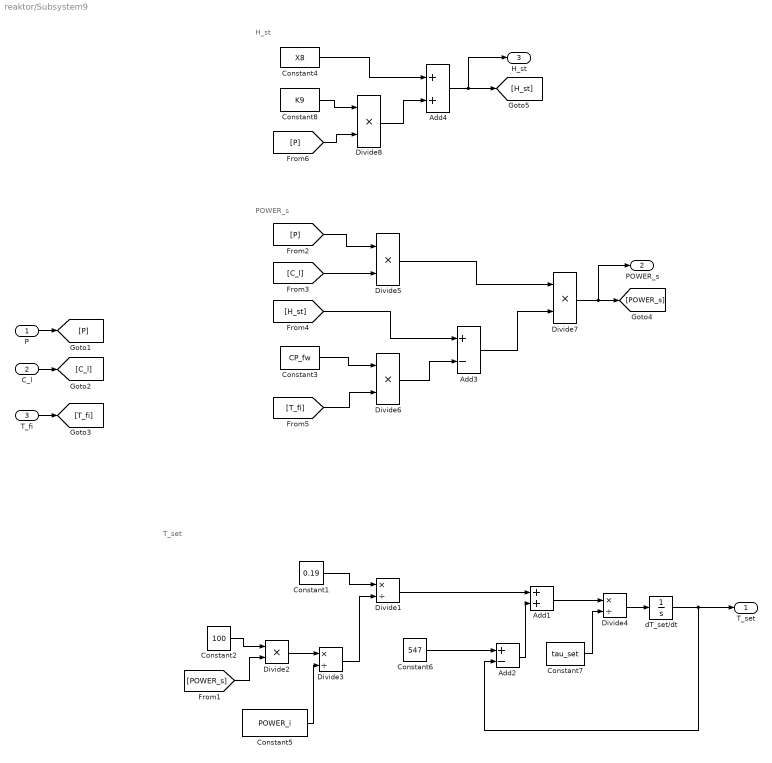
== system reaktor/Subsystem9 ==
  note: H_st
  note: POWER_s
  note: T_set
  P : Inport
  C_l : Inport  Port=2
  T_fi : Inport  Port=3
  Add1 : Sum
  Add2 : Sum  Inputs=+-
  Add3 : Sum  Inputs=+-
  Add4 : Sum  Inputs=2
  Constant1 : Constant  Value=0.19
  Constant2 : Constant  Value=100
  Constant3 : Constant  Value=CP_fw
  Constant4 : Constant  Value=X8
  Constant5 : Constant  Value=POWER_i
  Constant6 : Constant  Value=547
  Constant7 : Constant  Value=tau_set
  Constant8 : Constant  Value=K9
  Divide1 : Product  Inputs=*/
  Divide2 : Product  Inputs=**
  Divide3 : Product  Inputs=*/
  Divide4 : Product  Inputs=*/
  Divide{5..8} (4 alike) : Product
  dT_set/dt : Integrator  InitialCondition=566
  T_set : Outport
  POWER_s : Outport  Port=2
  H_st : Outport  Port=3
  wires:
  Constant1/1 -> Divide1/1
  Constant2/1 -> Divide2/1
  Divide2/1 -> Divide3/1
  Constant5/1 -> Divide3/2
  Divide3/1 -> Divide1/2
  Divide1/1 -> Add1/1
  Constant6/1 -> Add2/1
  Add2/1 -> Add1/2
  dT_set/dt/1 -> Add2/2, T_set/1
  Add1/1 -> Divide4/1
  Divide4/1 -> dT_set/dt/1
  Constant7/1 -> Divide4/2
  [POWER_s] -> Divide2/2
  P/1 -> [P]
  C_l/1 -> [C_l]
  T_fi/1 -> [T_fi]
  [C_l] -> Divide5/2
  [P] -> Divide5/1
  [T_fi] -> Divide6/2
  Constant3/1 -> Divide6/1
  [H_st] -> Add3/1
  Divide6/1 -> Add3/2
  Divide5/1 -> Divide7/1
  Add3/1 -> Divide7/2
  Divide7/1 -> POWER_s/1, [POWER_s]
  Constant8/1 -> Divide8/1
  [P] -> Divide8/2
  Constant4/1 -> Add4/1
  Divide8/1 -> Add4/2
  Add4/1 -> H_st/1, [H_st]

== matlab function reaktor/Subsystem11/MATLAB Function1 ==
  data: u input; y output
function y = fcn(u)
%#codegen

Roh = u;
y = (Roh*100)/0.00689;

== matlab function reaktor/Subsystem11/MATLAB Function ==
  data: u1 input; y1 output; u2 input; y2 output
function [y1,y2] = fcn(u1,u2)
%#codegen
%u1 = T_set
%u2 = T_aves

e = u1 - u2;

y2 = e;

R = 0.003375;

 if e > 5
     y1 = (72 * R * 0.00689) / 60;
 elseif e > 3 && e < 5
     y1 = (R * 0.00689 * (32 * (u1-u2) - 88)) / 60;
 elseif e > 1 && e > 3
     y1 = (8 * R * 0.00689) / 60;
 elseif e < 1 && e > -1
     y1 = 0;
 elseif e > -3 && e < -1
     y1 = (-8 * R * 0.00689) / 60;
 elseif e > -5 && e < -3
     y1 = (R * 0.00689 * (32 * (u1-u2) - 88)) / 60;
 else 
     y1 = (-72 * R * 0.00689) / 60;
 end
